simulink model "CommutationSimv2"  (Simulink 8.3)
settings: Solver=FixedStepDiscrete  StartTime=0.0  StopTime=1  FixedStep=.00001  RelTol=1e-3
undefined symbols (not defined in the file): abc, alphabeta, DiscIntNeverNeededParam, dq, MicrochipMotorControlTools, to
libraries: simulink x7
settings Model: Creator=Marx  LastModifiedBy=pavlo
settings DataIOCC: LimitDataPoints=off  SignalLoggingSaveFormat=Dataset
settings OptimizationCC: ExpressionDepthLimit=2147483647

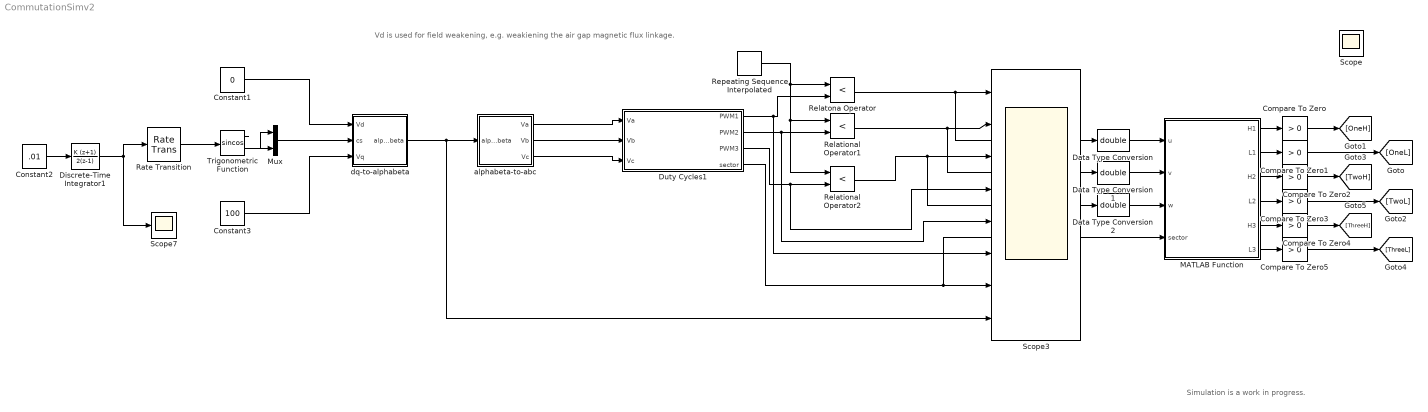
== system CommutationSimv2 ==
  note: Vd is used for field weakening, e.g. weakiening the air gap magnetic flux linkage.
  note: Simulation is a work in progress.
  Compare To Zero{,1..5} (6 alike) : simulink/Logic and Bit Operations/Compare To Zero  relop=>  OutDataTypeStr=boolean
  Constant1 : Constant  Value=0
  Constant2 : Constant  Value=.01
  Constant3 : Constant  Value=100
  Data Type Conversion : DataTypeConversion  OutDataTypeStr=double
  Data Type Conversion1 : DataTypeConversion  OutDataTypeStr=double
  Data Type Conversion2 : DataTypeConversion  OutDataTypeStr=double
  Discrete-Time Integrator1 : DiscreteIntegrator  IntegratorMethod=Accumulation: Trapezoidal  SampleTime=.0001  ICPrevOutput=DiscIntNeverNeededParam  ICPrevScaledInput=DiscIntNeverNeededParam
  Duty Cycles1 : MATLAB Function  TreatAsAtomicUnit=on
  MATLAB Function : MATLAB Function  TreatAsAtomicUnit=on
  Mux : Mux  Inputs=2
  Rate Transition : RateTransition  OutPortSampleTime=.00001
  Relational Operator1 : RelationalOperator  Operator=<  OutDataTypeStr=boolean
  Relational Operator2 : RelationalOperator  Operator=<  OutDataTypeStr=boolean
  Relatona Operator : RelationalOperator  Operator=<  OutDataTypeStr=boolean
  Repeating Sequence Interpolated : simulink/Sources/Repeating Sequence Interpolated  OutValues=[0 10000].'  TimeValues=[0 .001].'  LookUpMeth=Interpolation-Use End Values  tsamp=.00001  OutMin=[]  OutMax=[]  OutDataTypeStr=double  OutputDataTypeScalingMode=double  OutDataType=fixdt(0,8)  OutScaling=2^-10
  Scope : Scope
  Scope3 : Scope  NumInputPorts=8
      settings: YMin=-0.2~-0.2~-0.2~-20~-20~-20~-1~-100  YMax=1.2~1.2~1.2~10020~10020~10020~8~100  MaxDataPoints=500000
  Scope7 : Scope
      settings: YMin=0  YMax=9500  SaveName=ScopeData8
  Trigonometric Function : Trigonometry  Operator=sincos
  alphabeta-to-abc : Subsystem  AncestorBlock=MicrochipMotorControlTools/alphabeta-to-abc
  dq-to-alphabeta : Subsystem  AncestorBlock=MicrochipMotorControlTools/dq-to-alphabeta
  wires:
  Discrete-Time Integrator1/1 -> Scope7/1, Rate Transition/1
  Constant2/1 -> Discrete-Time Integrator1/1
  Mux/1 -> dq-to-alphabeta/2(cs)
  dq-to-alphabeta/1(alphabeta) -> alphabeta-to-abc/1(alphabeta), Scope3/8
  alphabeta-to-abc/1(Va) -> Duty Cycles1/1(Va)
  alphabeta-to-abc/2(Vb) -> Duty Cycles1/2(Vb)
  alphabeta-to-abc/3(Vc) -> Duty Cycles1/3(Vc)
  Constant1/1 -> dq-to-alphabeta/1(Vd)
  Constant3/1 -> dq-to-alphabeta/3(Vq)
  Trigonometric Function/2 -> Mux/1
  Trigonometric Function/1 -> Mux/2
  Duty Cycles1/1(PWM1) -> Relatona Operator/2, Scope3/6
  Duty Cycles1/2(PWM2) -> Relational Operator1/2, Scope3/5
  Duty Cycles1/3(PWM3) -> Relational Operator2/2, Scope3/4
  Repeating Sequence Interpolated/1 -> Relatona Operator/1, Relational Operator2/1, Relational Operator1/1
  Rate Transition/1 -> Trigonometric Function/1
  Relatona Operator/1 -> Data Type Conversion/1, Scope3/1
  Relational Operator1/1 -> Data Type Conversion1/1, Scope3/2
  Relational Operator2/1 -> Data Type Conversion2/1, Scope3/3
  Duty Cycles1/4(sector) -> MATLAB Function/4(sector), Scope3/7
  MATLAB Function/1(H1) -> Compare To Zero/1
  MATLAB Function/2(L1) -> Compare To Zero1/1
  MATLAB Function/3(H2) -> Compare To Zero2/1
  MATLAB Function/4(L2) -> Compare To Zero3/1
  MATLAB Function/5(H3) -> Compare To Zero4/1
  MATLAB Function/6(L3) -> Compare To Zero5/1
  Compare To Zero/1 -> [OneH]
  Compare To Zero1/1 -> [OneL]
  Compare To Zero2/1 -> [TwoH]
  Compare To Zero3/1 -> [TwoL]
  Compare To Zero4/1 -> [ThreeH]
  Compare To Zero5/1 -> [ThreeL]
  Data Type Conversion1/1 -> MATLAB Function/2(v)
  Data Type Conversion/1 -> MATLAB Function/1(u)
  Data Type Conversion2/1 -> MATLAB Function/3(w)

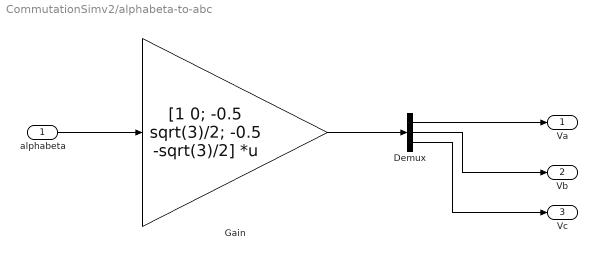
== system CommutationSimv2/alphabeta-to-abc ==
  alphabeta : Inport
  Demux : Demux  Outputs=3
  Gain : Gain  Gain=[1 0; -0.5 sqrt(3)/2; -0.5 -sqrt(3)/2]  Multiplication=Matrix(K*u)  OutDataTypeStr=single
  Va : Outport  OutDataTypeStr=single
  Vb : Outport  Port=2  OutDataTypeStr=single
  Vc : Outport  Port=3  OutDataTypeStr=single
  wires:
  alphabeta/1 -> Gain/1
  Gain/1 -> Demux/1
  Demux/1 -> Va/1
  Demux/2 -> Vb/1
  Demux/3 -> Vc/1

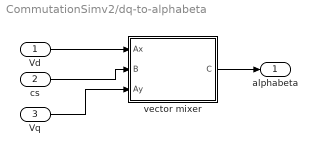
== system CommutationSimv2/dq-to-alphabeta ==
  Vd : Inport
  cs : Inport  Port=2
  Vq : Inport  Port=3
  vector mixer : Subsystem  AncestorBlock=MicrochipMotorControlTools/vector mixer
  alphabeta : Outport
  wires:
  cs/1 -> vector mixer/2(B)
  Vd/1 -> vector mixer/1(Ax)
  vector mixer/1(C) -> alphabeta/1
  Vq/1 -> vector mixer/3(Ay)

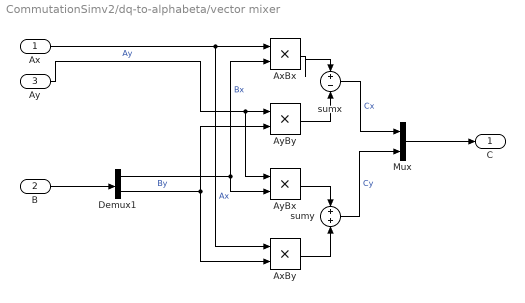
== system CommutationSimv2/dq-to-alphabeta/vector mixer ==
  Ax : Inport
  B : Inport  Port=2
  Ay : Inport  Port=3
  AxBx : Product  RndMeth=Zero  OutDataTypeStr=Inherit: Same as first input
  AxBy : Product  RndMeth=Zero  OutDataTypeStr=Inherit: Same as first input
  AyBx : Product  RndMeth=Zero  OutDataTypeStr=Inherit: Same as first input
  AyBy : Product  RndMeth=Zero  OutDataTypeStr=Inherit: Same as first input
  Demux1 : Demux  Outputs=2
  Mux : Mux  Inputs=2
  sumx : Sum  Inputs=+|-
  sumy : Sum  Inputs=+|+
  C : Outport
  wires:
  sumx/1 -> Mux/1  "Cx"
  B/1 -> Demux1/1
  Demux1/1 -> AyBx/2, AxBx/2  "Bx"
  Demux1/2 -> AxBy/2, AyBy/2  "By"
  sumy/1 -> Mux/2  "Cy"
  AxBy/1 -> sumy/2
  AyBx/1 -> sumy/1
  AxBx/1 -> sumx/1
  AyBy/1 -> sumx/2
  Ay/1 -> AyBy/1, AyBx/1  "Ay"
  Ax/1 -> AxBy/1, AxBx/1  "Ax"
  Mux/1 -> C/1

== matlab function MATLAB Function ==
  data: u input double; H1 output double; v input double; w input double; sector input double; L1 output double; H2 output double; L2 output boolean; H3 output boolean; L3 output boolean
function [H1, L1, H2, L2, H3, L3] = fcn(u, v, w, sector)
%#codegen

    if (sector == 3)
        H1 = u;
        H2 = 0;
        H3 = 0;
        L1 = 0;
        L2 = u;
        L3 = u;
    elseif (sector == 1)
        H1 = u;
        H2 = v;
        H3 = 0;
        L1 = 0;
        L2 = 0;
        L3 = 1;
    elseif (sector == 5)
        H1 = 0;
        H2 = v;
        H3 = 0;
        L1 = v;
        L2 = 0;
        L3 = v;
    elseif (sector == 4)
        H1 = 0;
        H2 = v;
        H3 = w;
        L1 = 1;
        L2 = 0;
        L3 = 0;
    elseif (sector == 6)
        H1 = 0;
        H2 = 0;
        H3 = w;
        L1 = w;
        L2 = w;
        L3 = 0;
    else
        H1 = u;
        H2 = 0;
        H3 = w;
        L1 = 0;
        L2 = 1;
        L3 = 0;
    end
end

== matlab function Duty Cycles1 ==
  data: PWM1 output single; Va input single; PWM2 output single; PWM3 output single; sector output double; Vb input double; Vc input double
function [PWM1, PWM2, PWM3, sector]  = DutyCycleCalc(Va, Vb, Vc)
%#codegen
PWM = single(100);

Ta = single(0);

if (Va >= 0)
    if (Vb >= 0)
        %Sector 3, 0 - 60 Degrees
        T1 = Vb;
        T2 = Va;
    
        T1 = T1*PWM;
        T2 = T2*PWM;
        Tc = (PWM-T1-T2)/2;
        Tb = Ta + T1;
        Ta = Tb + T2;
    
        PWM1 = single(0);
        PWM2 = Tb;
        PWM3 = Ta;
        sector = single(3);
    else
        if (Vc >= 0)
           %Sector 5, 120 - 180 Degrees
            T1 = Va;
            T2 = Vc;
    
            T1 = T1*PWM;
            T2 = T2*PWM;
            Tc = (PWM-T1-T2)/2;
            Tb = Ta + T1;
            Ta = Tb + T2;
    
            PWM1 = Ta;
            PWM2 = single(0);
            PWM3 = Tb;
            sector = single(5);
        else
            %Sector 1, 60 - 120 Degrees
            T1 = -Vb;
            T2 = -Vc;
    
            T1 = T1*PWM;
            T2 = T2*PWM;
            Tc = (PWM-T1-T2)/2;
            Tb = Ta + T1;
            Ta = Tb + T2;
    
            PWM1 = Tb;
            PWM2 = single(0);
            PWM3 = Ta;
            sector = single(1);
        end
    end
else
    if (Vb >= 0)
        if (Vc >= 0)
            %Sector 6, 240 - 300 Degrees
            T1 = Vc;
            T2 = Vb;
    
            T1 = T1*PWM;
            T2 = T2*PWM;
            Tc = (PWM-T1-T2)/2;
            Tb = Ta + T1;
            Ta = Tb + T2;
    
            PWM1 = Tb;
            PWM2 = Ta;
            PWM3 = single(0);
            sector = single(6);
        else
            %Sector 2, 300 - 0 Degrees
            T1 = -Vc;
            T2 = -Va;
    
            T1 = T1*PWM;
            T2 = T2*PWM;
            Tc = (PWM-T1-T2)/2;
            Tb = Ta + T1;
            Ta = Tb + T2;
    
            PWM1 = single(0);
            PWM2 = Ta;
            PWM3 = Tb;
            sector = single(2);
        end
    else
        %Sector 4, 180 - 240 Degrees
        T1 = -Va;
        T2 = -Vb;
    
        T1 = T1*PWM;
        T2 = T2*PWM;
        Tc = (PWM-T1-T2)/2;
        Tb = Ta + T1;
        Ta = Tb + T2;
    
        PWM1 = Ta;
        PWM2 = Tb;
        PWM3 = single(0);
        sector = single(4);
    end
end

end
